simulink model "E5S_Prueba_Simulacion_Hibrido"  (R2020a)
settings: Solver=VariableStepAuto  StartTime=0.0  StopTime=0.5  RelTol=1e-3
undefined symbols (not defined in the file): J_a, K_hib
libraries: fl_lib x4, nesl_utility x4, ee_lib x3
settings Model: Creator=Luis Angel  LastModifiedBy=Luis Angel

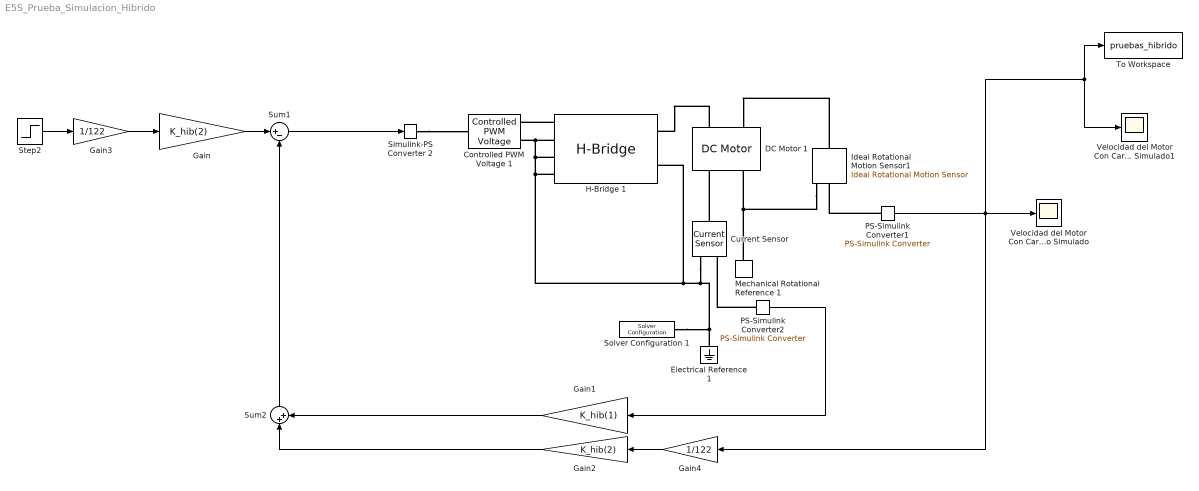
== system E5S_Prueba_Simulacion_Hibrido ==
  " Ideal Rotational Motion Sensor1" : fl_lib/Mechanical/Mechanical Sensors/Ideal Rotational Motion Sensor  wrap_angle=simscape.enum.onoff.off  offset=0 rad
  " PS-Simulink Converter1" : nesl_utility/PS-Simulink Converter  PhysicalDomain=network_engine_domain  SubClassName=ps_output  LeftPortType=input  RightPortType=output  PseudoPeriodic=off  Frequencies=[]  Unit=rad/s  AffineConversion=on
  " PS-Simulink Converter2" : nesl_utility/PS-Simulink Converter  PhysicalDomain=network_engine_domain  SubClassName=ps_output  LeftPortType=input  RightPortType=output  PseudoPeriodic=off  Frequencies=[]  Unit=A  AffineConversion=on
  Controlled PWM Voltage 1 : ee_lib/Integrated Circuits/Controlled PWM Voltage  F=1000 Hz  TD=0 s  pulse_width_offset=0 s  pulse_min=0 s  Vmin=0 V  Vmax=5 V  Vm=5 V  pwm_or_av=2  event_type=1  sample_time=1e-6 s  u_min=0  u_max=1
      settings: InternalSimscapePortConfiguration="{\"Bottom\":[],\"Left\":[{\"id\":\"u\",\"label\":\"u\",\"type\":\"input\"}],\"Right\":[{\"id\":\"p2\",\"label\":\"PWM\",\"type\":\"foundation.electrical.electrical\"},{\"id\":\"n2\",\"label\":\"REF\",\"type\":\"foundation.electrical.electrical\"}],\"Top\":[]}"
  Current Sensor : fl_lib/Electrical/Electrical Sensors/Current Sensor
  DC Motor 1 : ee_lib/Electromechanical/Brushed Motors/DC Motor  field_option=ee.enum.field_option.pm  Rf=100 Ohm  Lf=1 H  Laf=0.15 H  If0=0 A  parameterization=ee.enum.dcparam_option.circuit_param  Ra=R Ohm  La=L H  emf_or_torque=ee.enum.emf_or_torque.kv  Kv=km V/(rad/s)  Ki=6.876e-4 N*m/A  T_stall=0.24e-3 N*m  w_max=19100 rpm  w_rated=15000 rpm  P_rated=0.08 W  V_rated=1.5 V  J=J_a kg*m^2  lam_param=ee.enum.lam_param.damping  lam=B N*m/(rad/s)  i_noload=0 A  V_i_noload=1.5 V  speed0=0 rad/s  alpha=3.93e-3 1/K  Tmeas=25 degC  thermal_mass=100 J/K  initial_temperature=25 degC
  Electrical Reference 1 : fl_lib/Electrical/Electrical Elements/Electrical Reference
      settings: SourceProductBaseCode=MT,SS
  Gain : Gain  Gain=K_hib(2)
  Gain1 : Gain  Gain=K_hib(1)
  Gain2 : Gain  Gain=K_hib(2)
  Gain3 : Gain  Gain=1/122
  Gain4 : Gain  Gain=1/122
  H-Bridge 1 : ee_lib/Semiconductors & Converters/Converters/H-Bridge  supply_ports=ee.enum.supply_ports.hidesupply  Venable=2.5 V  Vmax=5 V  Vreverse=2.5 V  Vbrake=2.5 V  Vm=Va V  pwm_or_av=ee.enum.pwm_or_av.averaged  regenerative_braking_mode=ee.enum.converters.regenerative_braking_mode.always_enabled  discontinuous=ee.enum.current_profile.continuous  freewheeling_mode=ee.enum.converters.freewheeling_mode.one_switch_one_diode  Ron=0.1 Ohm  Don=0.05 Ohm  Goff=1e-6 S  Rload=10 Ohm  Lload=1e-5 H  F=10 kHz  thermal_mass=100 J/K  initial_temperature=298.15 K  Ron2=0.1 Ohm  Don2=0.05 Ohm  Tmeas=298.15 K  Tmeas2=398.15 K
  Mechanical Rotational Reference 1 : fl_lib/Mechanical/Rotational Elements/Mechanical Rotational Reference
  Simulink-PS Converter 2 : nesl_utility/Simulink-PS Converter  PhysicalDomain=network_engine_domain  SubClassName=ps_input  LeftPortType=input  RightPortType=output  PseudoPeriodic=off  Frequencies=[]  NoiseDistribution=none  NoiseParameters=[]  Unit=1  AffineConversion=off  FilteringAndDerivatives=provide  SimscapeFilterOrder=1  InputFilterTimeConstant=0.001  UdotUserProvided=0
  Solver Configuration 1 : nesl_utility/Solver Configuration  PhysicalDomain=network_engine_domain  SubClassName=solver  LeftPortType=input  RightPortType=generic  Tones=[]  Harmonics=[]  SimulateNoise=off  Profile=off  UseLocalSampling=off  EnableSwitchedLinearOptims=on  FrequencyDomain=off  UseCCode=off  RelTol=0.001  AbsTol=1e-06  MinStep=1e-09  ToWorkspace=off  RevertToSquareIcSolve=off  NumHomotopyIterations=100  PhasorMode=off  PhasorModeNumHarmonics=1  DoDC=off  ResidualTolerance=1e-09  UseLocalSolver=off  LocalSolverChoice=NE_BACKWARD_EULER_ADVANCER  LocalSolverSampleTime=0.001  DoFixedCost=off  MaxNonlinIter=3  MaxModeIter=2  LinearAlgebra=auto  EquationFormulation=NE_TIME_EF  DelaysMemoryBudget=1024  AutomaticFiltering=on  FilteringTimeConstant=0.001  PartitionStorageMethod=AS_NEEDED  PartitionMemoryBudget=1024  PartitionMethod=ROBUST
  Step2 : Step  Time=0  After=52.46  SampleTime=0
  Sum1 : Sum  Inputs=|+-
  Sum2 : Sum  Inputs=|++
  To Workspace : ToWorkspace  VariableName=pruebas_hibrido  SaveFormat=Timeseries  SampleTime=0.00001
  Velocidad del Motor Con Carga Controlado Simulado : Scope
  Velocidad del Motor Con Carga Controlado Simulado1 : Scope
  wires:
  Gain4/1 -> Gain2/1
  Gain3/1 -> Gain/1
  Sum2/1 -> Sum1/2
  Gain/1 -> Sum1/1
  Sum1/1 -> Simulink-PS Converter 2/1
  Step2/1 -> Gain3/1
  Gain1/1 -> Sum2/2
  " PS-Simulink Converter2"/1 -> Gain1/1
  Gain2/1 -> Sum2/1
  " PS-Simulink Converter1"/1 -> Velocidad del Motor Con Carga Controlado Simulado1/1, To Workspace/1, Gain4/1, Velocidad del Motor Con Carga Controlado Simulado/1
  connections:
  Mechanical Rotational Reference 1/LConn1 -- " Ideal Rotational Motion Sensor1"/RConn1 -- DC Motor 1/RConn2
  Controlled PWM Voltage 1/RConn2 -- H-Bridge 1/RConn2 -- Solver Configuration 1/RConn1 -- Electrical Reference 1/LConn1 -- Current Sensor/RConn2 -- H-Bridge 1/LConn4 -- H-Bridge 1/LConn3 -- H-Bridge 1/LConn2
  Current Sensor/LConn1 -- DC Motor 1/RConn1
  H-Bridge 1/LConn1 -- Controlled PWM Voltage 1/RConn1
  " PS-Simulink Converter1"/LConn1 -- " Ideal Rotational Motion Sensor1"/RConn2
  Simulink-PS Converter 2/RConn1 -- Controlled PWM Voltage 1/LConn1
  " Ideal Rotational Motion Sensor1"/LConn1 -- DC Motor 1/LConn2
  " PS-Simulink Converter2"/LConn1 -- Current Sensor/RConn1
  DC Motor 1/LConn1 -- H-Bridge 1/RConn1
